simulink library "Lib_Turbo_Shaft_TMATS"  (Simulink 8.5)
settings: Solver=ode45  StartTime=0.0  StopTime=10.0  RelTol=1e-3
Description:
  | Thomas Modules
settings Model: Creator=jwchapm2  LastModifiedBy=jwchapm2

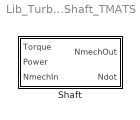
== system Lib_Turbo_Shaft_TMATS ==
  Shaft : Subsystem  mask(T-MATS: Shaft Library Block){Shaft_Inertia_M=0.3183}
      mask prompts: Shaft_Inertia_M "Shaft_Inertia_M - Shaft Inertia Term [slugs*ft2]"
      mask help: This block simulates the performance of a shaft using basic dynamic equations and properties.
      mask Help: web(which('Turbo_TMATS_Shft.html'),'-helpbrowser')

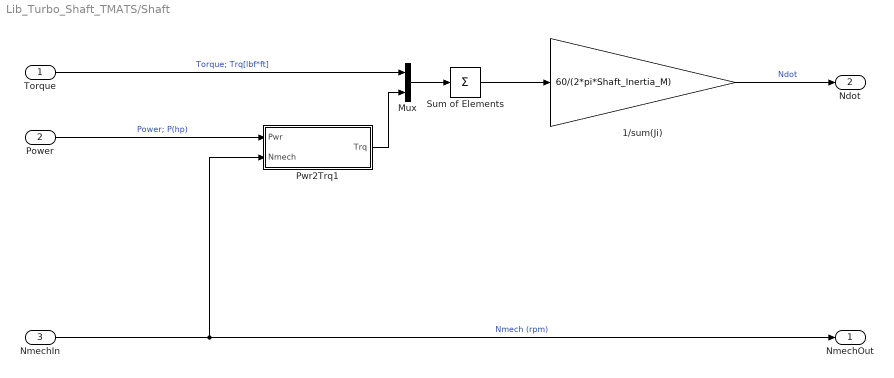
== system Lib_Turbo_Shaft_TMATS/Shaft ==
  Torque : Inport
  Power : Inport  Port=2
  NmechIn : Inport  Port=3
  1/sum(Ji) : Gain  Gain=60/(2*pi*Shaft_Inertia_M)  SaturateOnIntegerOverflow=on  OutDataTypeStr=Inherit: Same as input  ParamDataTypeStr=Inherit: Same as input
  Mux : Mux  Inputs=2
  Pwr2Trq1 : Subsystem
  Sum of Elements : Sum  Inputs=+
  NmechOut : Outport
  Ndot : Outport  Port=2
  wires:
  NmechIn/1 -> Pwr2Trq1/2(Nmech), NmechOut/1  "Nmech (rpm)"
  1/sum(Ji)/1 -> Ndot/1  "Ndot"
  Torque/1 -> Mux/1  "Torque; Trq[lbf*ft]"
  Sum of Elements/1 -> 1/sum(Ji)/1
  Mux/1 -> Sum of Elements/1
  Pwr2Trq1/1(Trq) -> Mux/2
  Power/1 -> Pwr2Trq1/1(Pwr)  "Power; P(hp)"

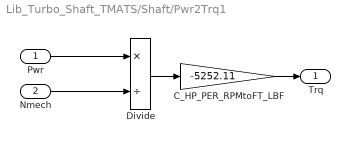
== system Lib_Turbo_Shaft_TMATS/Shaft/Pwr2Trq1 ==
  Pwr : Inport
  Nmech : Inport  Port=2
  C_HP_PER_RPMtoFT_LBF : Gain  Gain=-5252.11
  Divide : Product  Inputs=*/
  Trq : Outport
  wires:
  Pwr/1 -> Divide/1
  Divide/1 -> C_HP_PER_RPMtoFT_LBF/1
  C_HP_PER_RPMtoFT_LBF/1 -> Trq/1
  Nmech/1 -> Divide/2
